simulink model "full_r2019b"  (R2019b)
settings: Solver=VariableStepAuto  StartTime=0.0  StopTime=10.0  RelTol=1e-3
settings Model: Creator=decla  LastModifiedBy=decla

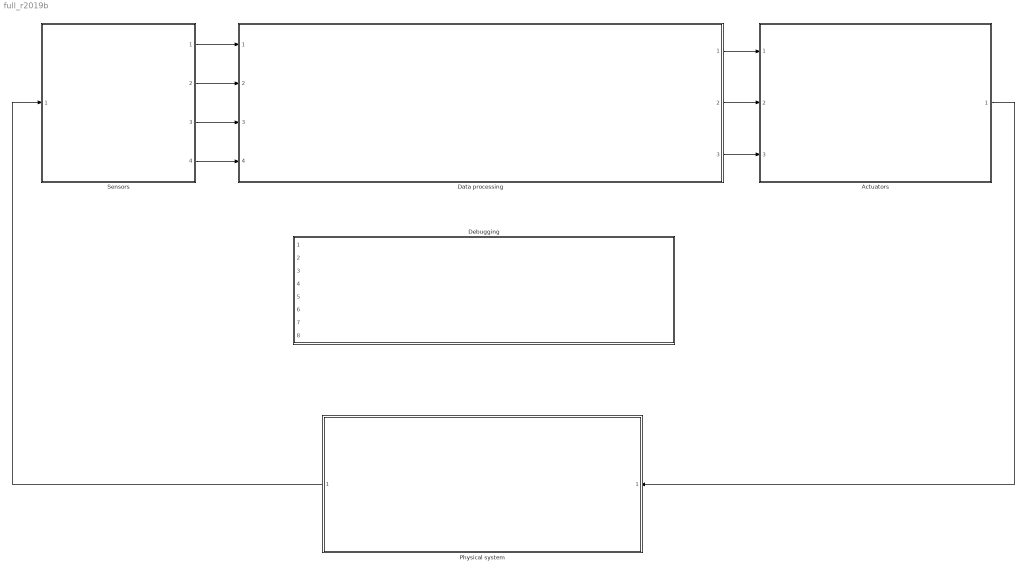
== system full_r2019b ==
  Actuators : Subsystem  ReferencedSubsystem=Actuators
  Data processing : Subsystem  ReferencedSubsystem=Data_processing
  Debugging : Subsystem  ReferencedSubsystem=Debugging
  Physical system : Subsystem  ReferencedSubsystem=Physical_system
  Sensors : Subsystem  ReferencedSubsystem=Sensors
  wires:
  Data processing/3 -> Actuators/3
  Actuators/1 -> Physical system/1
  Physical system/1 -> Sensors/1
  Sensors/4 -> Data processing/4
  Sensors/3 -> Data processing/3
  Sensors/2 -> Data processing/2
  Sensors/1 -> Data processing/1
  Data processing/2 -> Actuators/2
  Data processing/1 -> Actuators/1
